simulink subsystem "Sensors"  (R2025b)
settings: Solver=VariableStepAuto  StartTime=0.0  StopTime=10.0  RelTol=1e-3
settings Model: Creator=joedo  LastModifiedBy=finnb

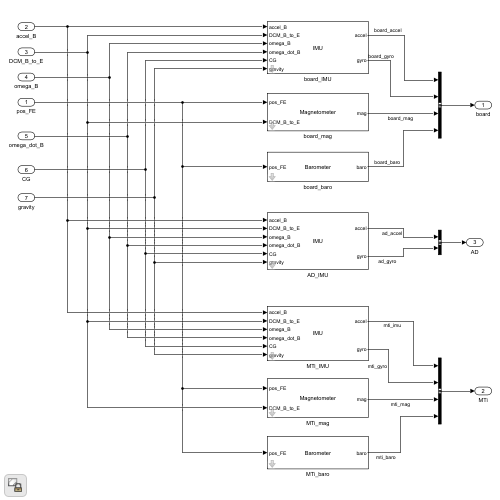
[thumbnail: Simulink's stored preview of the top-level diagram]
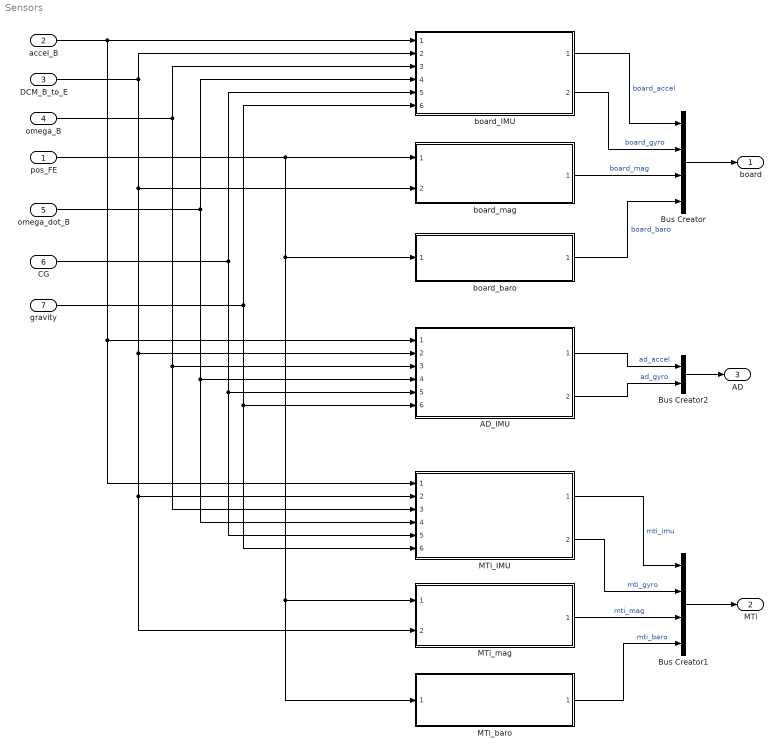
== system Sensors ==
  pos_FE : Inport
  accel_B : Inport  Port=2
  DCM_B_to_E : Inport  Port=3
  omega_B : Inport  Port=4
  omega_dot_B : Inport  Port=5
  CG : Inport  Port=6
  gravity : Inport  Port=7
  AD_IMU : Subsystem  ReferencedSubsystem=sensor_IMU  samplingrate=200  noise_accel=[1,1,1]*1e-3  bias_accel=[0 0 0]  scale_accel=[1 0 0; 0 1 0; 0 0 1]  lim_accel=inf  noise_gyro=[1,1,1]*1e-9  bias_gyro=[0 0 0]  scale_gyro=[1 0 0; 0 1 0; 0 0 1]  lim_gyro=inf  S=[1 0 0; 0 1 0; 0 0 1]  d=[0 0 0]
  Bus Creator : BusCreator  Inputs=4
  Bus Creator1 : BusCreator  Inputs=4
  Bus Creator2 : BusCreator  Inputs=2
  MTi_IMU : Subsystem  ReferencedSubsystem=sensor_IMU  samplingrate=200  noise_accel=[1,1,1]*1e-3  bias_accel=[0 0 0]  scale_accel=[1 0 0; 0 1 0; 0 0 1]  lim_accel=inf  noise_gyro=[1,1,1]*1e-9  bias_gyro=[0 0 0]  scale_gyro=[1 0 0; 0 1 0; 0 0 1]  lim_gyro=inf  S=[1 0 0; 0 1 0; 0 0 1]  d=[0 0 0]
  MTi_baro : Subsystem  ReferencedSubsystem=sensor_baro  samplingrate=100  noise_pres=0.2  bias_pres=0  scale_pres=1  limit_pres=[0, inf]
  MTi_mag : Subsystem  ReferencedSubsystem=sensor_mag  samplingrate=100  noise_mag=[1,1,1]*1e-2  bias_mag=[0 0 0]  scale_mag=[1 0 0; 0 1 0; 0 0 1]  limit_mag=0  Ssi=[1 0 0; 0 1 0; 0 0 1]  Lsi=[0 0 0]  lon=80.5204  lat=43.4643  year=2025
  board_IMU : Subsystem  ReferencedSubsystem=sensor_IMU  samplingrate=200  noise_accel=[1,1,1]*1e-3  bias_accel=[0 0 0]  scale_accel=[1 0 0; 0 1 0; 0 0 1]  lim_accel=inf  noise_gyro=[1,1,1]*1e-9  bias_gyro=[0 0 0]  scale_gyro=[1 0 0; 0 1 0; 0 0 1]  lim_gyro=inf  S=[1 0 0; 0 1 0; 0 0 1]  d=[0 0 0]
  board_baro : Subsystem  ReferencedSubsystem=sensor_baro  samplingrate=100  noise_pres=0.2  bias_pres=0  scale_pres=1  limit_pres=[0, inf]
  board_mag : Subsystem  ReferencedSubsystem=sensor_mag  samplingrate=100  noise_mag=[1,1,1]*1e-2  bias_mag=[0 0 0]  scale_mag=[1 0 0; 0 1 0; 0 0 1]  limit_mag=0  Ssi=[1 0 0; 0 1 0; 0 0 1]  Lsi=[0 0 0]  lon=80.5204  lat=43.4643  year=2025
  board : Outport
  MTi : Outport  Port=2
  AD : Outport  Port=3
  wires:
  Bus Creator/1 -> board/1
  board_baro/1 -> Bus Creator/4  "board_baro"
  MTi_baro/1 -> Bus Creator1/4  "mti_baro"
  MTi_IMU/1 -> Bus Creator1/1  "mti_imu"
  MTi_mag/1 -> Bus Creator1/3  "mti_mag"
  Bus Creator1/1 -> MTi/1
  AD_IMU/1 -> Bus Creator2/1  "ad_accel"
  Bus Creator2/1 -> AD/1
  pos_FE/1 -> MTi_baro/1, MTi_mag/1, board_baro/1, board_mag/1
  DCM_B_to_E/1 -> board_IMU/2, MTi_mag/2, MTi_IMU/2, AD_IMU/2, board_mag/2
  accel_B/1 -> MTi_IMU/1, AD_IMU/1, board_IMU/1
  omega_B/1 -> MTi_IMU/3, AD_IMU/3, board_IMU/3
  omega_dot_B/1 -> MTi_IMU/4, AD_IMU/4, board_IMU/4
  CG/1 -> MTi_IMU/5, AD_IMU/5, board_IMU/5
  gravity/1 -> MTi_IMU/6, AD_IMU/6, board_IMU/6
  AD_IMU/2 -> Bus Creator2/2  "ad_gyro"
  MTi_IMU/2 -> Bus Creator1/2  "mti_gyro"
  board_IMU/1 -> Bus Creator/1  "board_accel"
  board_IMU/2 -> Bus Creator/2  "board_gyro"
  board_mag/1 -> Bus Creator/3  "board_mag"
